simulink subsystem "NAVIGATION"  (R2025b)
settings: Solver=VariableStepAuto  StartTime=0.0  StopTime=10.0  RelTol=1e-3
model mask{refTimePosix=0, omgCelBod=0}
  mask prompts: refTimePosix "Reference time for ECI2ECEF conversion (UTC, Posix) [s]"; omgCelBod "Celestial body angular velocity [rads-1]"
undefined symbols (not defined in the file): simData
libraries: simulink_extras x4, simulink x3, matrix_library x2, aerolibtransform2 x2
settings Model: Creator=antoniohernandez-rodiciomateos  LastModifiedBy=antoniohernandez-rodiciomateos

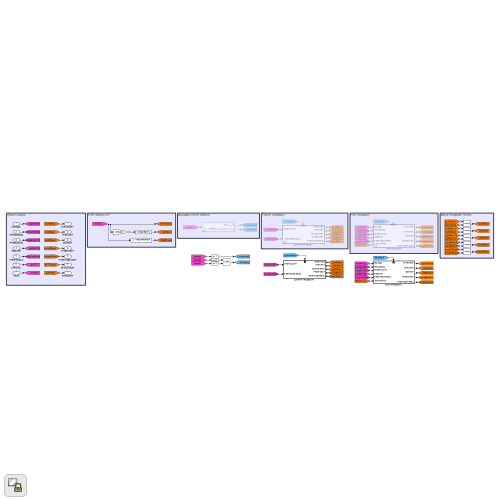
[thumbnail: Simulink's stored preview of the top-level diagram]
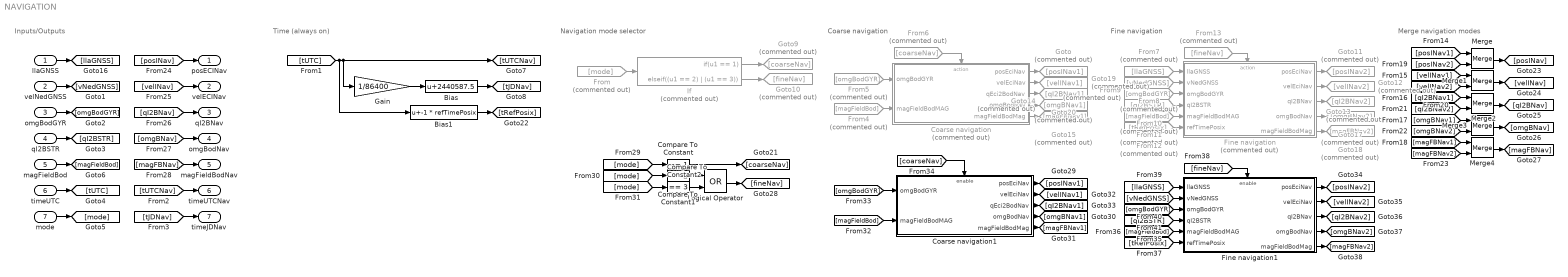
== system NAVIGATION ==
  note: Inputs/Outputs
  note: Time (always on)
  note: Navigation mode selector
  note: Coarse navigation
  note: Fine navigation
  note: Merge navigation modes
  llaGNSS : Inport  PortDimensions=[3 1]
  velNedGNSS : Inport  Port=2  PortDimensions=[3 1]
  omgBodGYR : Inport  Port=3  PortDimensions=[3 1]
  qI2BSTR : Inport  Port=4  PortDimensions=[4 1]
  magFieldBod : Inport  Port=5  PortDimensions=[3 1]
  timeUTC : Inport  Port=6  PortDimensions=[1 1]
  mode : Inport  Port=7  PortDimensions=[1 1]
  Bias : Bias  Bias=2440587.5  SaturateOnIntegerOverflow=off
  Bias1 : Bias  Bias=-1 * refTimePosix  SaturateOnIntegerOverflow=off
  Coarse navigation : Subsystem  Commented=on  TreatAsAtomicUnit=on
  Coarse navigation1 : Subsystem  TreatAsAtomicUnit=on
  Compare To Constant : simulink/Logic and Bit Operations/Compare To Constant  relop===  const=1  OutDataTypeStr=boolean
  Compare To Constant1 : simulink/Logic and Bit Operations/Compare To Constant  relop===  const=2  OutDataTypeStr=boolean
  Compare To Constant2 : simulink/Logic and Bit Operations/Compare To Constant  relop===  const=3  OutDataTypeStr=boolean
  Fine navigation : Subsystem  Commented=on  TreatAsAtomicUnit=on
  Fine navigation1 : Subsystem  TreatAsAtomicUnit=on
  From : From  Commented=on  GotoTag=mode
  From10 : From  Commented=on  GotoTag=qI2BSTR
  From11 : From  Commented=on  GotoTag=magFieldBod
  From12 : From  Commented=on  GotoTag=tRefPosix
  From13 : From  Commented=on  GotoTag=fineNav
  From4 : From  Commented=on  GotoTag=magFieldBod
  From5 : From  Commented=on  GotoTag=omgBodGYR
  From6 : From  Commented=on  GotoTag=coarseNav
  From7 : From  Commented=on  GotoTag=llaGNSS
  From8 : From  Commented=on  GotoTag=vNedGNSS
  From9 : From  Commented=on  GotoTag=omgBodGYR
  Gain : Gain  Gain=1/86400
  Goto : Goto  Commented=on  GotoTag=posINav1
  Goto10 : Goto  Commented=on  GotoTag=fineNav
  Goto11 : Goto  Commented=on  GotoTag=posINav2
  Goto12 : Goto  Commented=on  GotoTag=velINav2
  Goto13 : Goto  Commented=on  GotoTag=qI2BNav2
  Goto14 : Goto  Commented=on  GotoTag=omgBNav1
  Goto15 : Goto  Commented=on  GotoTag=magFBNav1
  Goto17 : Goto  Commented=on  GotoTag=omgBNav2
  Goto18 : Goto  Commented=on  GotoTag=magFBNav2
  Goto19 : Goto  Commented=on  GotoTag=velINav1
  Goto20 : Goto  Commented=on  GotoTag=qI2BNav1
  Goto9 : Goto  Commented=on  GotoTag=coarseNav
  If : If  Commented=on  IfExpression=u1 == 1  ElseIfExpressions=(u1 == 2) | (u1 == 3)  ShowElse=off
  Logical Operator : Logic  Operator=OR  AllPortsSameDT=off  OutDataTypeStr=boolean
  Merge{,1..4} (5 alike) : Merge
  posECINav : Outport  PortDimensions=[3 1]
  velECINav : Outport  Port=2  PortDimensions=[3 1]
  qI2BNav : Outport  Port=3  PortDimensions=[4 1]
  omgBodNav : Outport  Port=4  PortDimensions=[3 1]
  magFieldBodNav : Outport  Port=5  PortDimensions=[3 1]
  timeUTCNav : Outport  Port=6  PortDimensions=[1 1]
  timeJDNav : Outport  Port=7  PortDimensions=[1 1]
  wires:
  llaGNSS/1 -> [llaGNSS]
  velNedGNSS/1 -> [vNedGNSS]
  omgBodGYR/1 -> [omgBodGYR]
  qI2BSTR/1 -> [qI2BSTR]
  timeUTC/1 -> [tUTC]
  mode/1 -> [mode]
  From/1 -> If/1
  magFieldBod/1 -> [magFieldBod]
  [tUTC] -> Bias1/1, Gain/1, [tUTCNav]
  Gain/1 -> Bias/1
  Bias/1 -> [tJDNav]
  [tUTCNav] -> timeUTCNav/1
  [tJDNav] -> timeJDNav/1
  If/1 -> Goto9/1
  If/2 -> Goto10/1
  Bias1/1 -> [tRefPosix]
  [posINav] -> posECINav/1
  [velINav] -> velECINav/1
  [qI2BNav] -> qI2BNav/1
  [omgBNav] -> omgBodNav/1
  [magFBNav] -> magFieldBodNav/1
  From6/1 -> Coarse navigation/Action
  Coarse navigation/2(velEciNav) -> Goto19/1
  Coarse navigation/4(omgBodNav) -> Goto14/1
  Coarse navigation/3(qEci2BodNav) -> Goto20/1
  Coarse navigation/1(posEciNav) -> Goto/1
  Coarse navigation/5(magFieldBodMag) -> Goto15/1
  From5/1 -> Coarse navigation/1(omgBodGYR)
  From4/1 -> Coarse navigation/2(magFieldBodMAG)
  Fine navigation/1(posEciNav) -> Goto11/1
  From10/1 -> Fine navigation/4(qI2BSTR)
  From13/1 -> Fine navigation/Action
  Fine navigation/3(qI2BNav) -> Goto13/1
  Fine navigation/5(magFieldBodMag) -> Goto18/1
  From7/1 -> Fine navigation/1(llaGNSS)
  Fine navigation/4(omgBodNav) -> Goto17/1
  From11/1 -> Fine navigation/5(magFieldBodMAG)
  Fine navigation/2(velEciNav) -> Goto12/1
  From8/1 -> Fine navigation/2(vNedGNSS)
  From9/1 -> Fine navigation/3(omgBodGYR)
  From12/1 -> Fine navigation/6(refTimePosix)
  [qI2BNav2] -> Merge2/2
  Merge2/1 -> [qI2BNav]
  Merge4/1 -> [magFBNav]
  [omgBNav2] -> Merge3/2
  Merge3/1 -> [omgBNav]
  [omgBNav1] -> Merge3/1
  [posINav1] -> Merge/1
  [velINav1] -> Merge1/1
  Merge/1 -> [posINav]
  [velINav2] -> Merge1/2
  [posINav2] -> Merge/2
  [magFBNav1] -> Merge4/1
  [magFBNav2] -> Merge4/2
  Merge1/1 -> [velINav]
  [qI2BNav1] -> Merge2/1
  [mode] -> Compare To Constant/1
  Compare To Constant/1 -> [coarseNav]
  [mode] -> Compare To Constant1/1
  [mode] -> Compare To Constant2/1
  Compare To Constant1/1 -> Logical Operator/1
  Compare To Constant2/1 -> Logical Operator/2
  Logical Operator/1 -> [fineNav]
  Coarse navigation1/1(posEciNav) -> [posINav1]
  Coarse navigation1/2(velEciNav) -> [velINav1]
  Coarse navigation1/3(qEci2BodNav) -> [qI2BNav1]
  Coarse navigation1/4(omgBodNav) -> [omgBNav1]
  Coarse navigation1/5(magFieldBodMag) -> [magFBNav1]
  [omgBodGYR] -> Coarse navigation1/1(omgBodGYR)
  [magFieldBod] -> Coarse navigation1/2(magFieldBodMAG)
  [coarseNav] -> Coarse navigation1/Enable
  [tRefPosix] -> Fine navigation1/6(refTimePosix)
  [qI2BSTR] -> Fine navigation1/4(qI2BSTR)
  Fine navigation1/2(velEciNav) -> [velINav2]
  Fine navigation1/5(magFieldBodMag) -> [magFBNav2]
  Fine navigation1/1(posEciNav) -> [posINav2]
  [magFieldBod] -> Fine navigation1/5(magFieldBodMAG)
  [vNedGNSS] -> Fine navigation1/2(vNedGNSS)
  [fineNav] -> Fine navigation1/Enable
  [llaGNSS] -> Fine navigation1/1(llaGNSS)
  Fine navigation1/3(qI2BNav) -> [qI2BNav2]
  [omgBodGYR] -> Fine navigation1/3(omgBodGYR)
  Fine navigation1/4(omgBodNav) -> [omgBNav2]

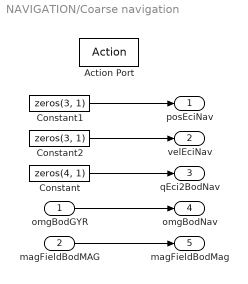
== system NAVIGATION/Coarse navigation ==
  omgBodGYR : Inport  PortDimensions=[3 1]
  magFieldBodMAG : Inport  Port=2  PortDimensions=[3 1]
  Action Port : ActionPort
  Constant : Constant  Value=zeros(4, 1)
  Constant1 : Constant  Value=zeros(3, 1)
  Constant2 : Constant  Value=zeros(3, 1)
  posEciNav : Outport  PortDimensions=[3 1]
  velEciNav : Outport  Port=2  PortDimensions=[3 1]
  qEci2BodNav : Outport  Port=3  PortDimensions=[4 1]
  omgBodNav : Outport  Port=4  PortDimensions=[3 1]
  magFieldBodMag : Outport  Port=5  PortDimensions=[3 1]
  wires:
  omgBodGYR/1 -> omgBodNav/1
  magFieldBodMAG/1 -> magFieldBodMag/1
  Constant/1 -> qEci2BodNav/1
  Constant1/1 -> posEciNav/1
  Constant2/1 -> velEciNav/1

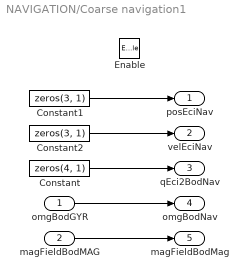
== system NAVIGATION/Coarse navigation1 ==
  omgBodGYR : Inport  PortDimensions=[3 1]
  magFieldBodMAG : Inport  Port=2  PortDimensions=[3 1]
  Enable : EnablePort
  Constant : Constant  Value=zeros(4, 1)
  Constant1 : Constant  Value=zeros(3, 1)
  Constant2 : Constant  Value=zeros(3, 1)
  posEciNav : Outport  PortDimensions=[3 1]
  velEciNav : Outport  Port=2  PortDimensions=[3 1]
  qEci2BodNav : Outport  Port=3  PortDimensions=[4 1]
  omgBodNav : Outport  Port=4  PortDimensions=[3 1]
  magFieldBodMag : Outport  Port=5  PortDimensions=[3 1]
  wires:
  omgBodGYR/1 -> omgBodNav/1
  magFieldBodMAG/1 -> magFieldBodMag/1
  Constant/1 -> qEci2BodNav/1
  Constant1/1 -> posEciNav/1
  Constant2/1 -> velEciNav/1

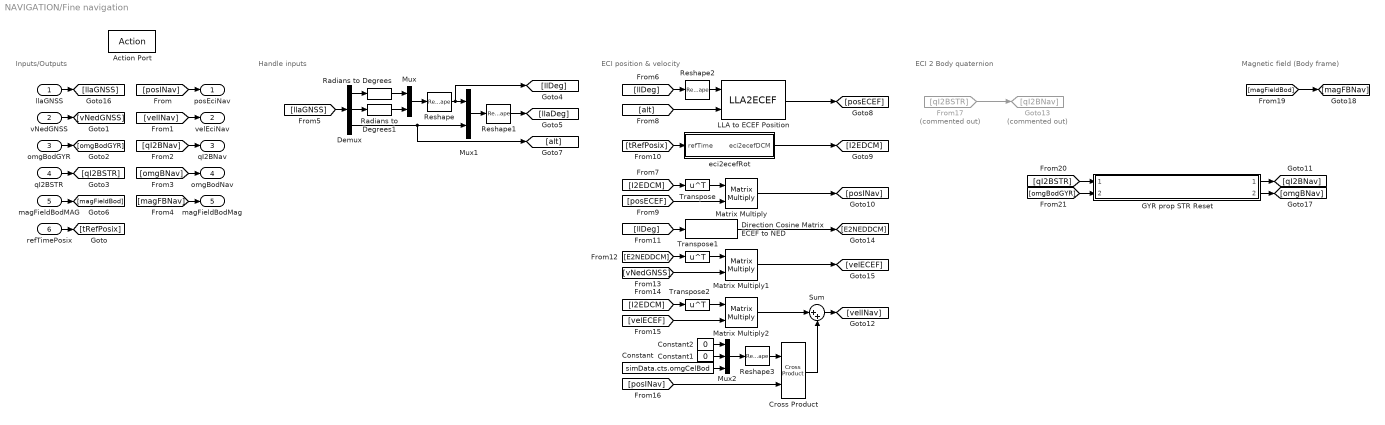
== system NAVIGATION/Fine navigation ==
  note: Inputs/Outputs
  note: Handle inputs
  note: ECI position & velocity
  note: ECI 2 Body quaternion
  note: Magnetic field (Body frame)
  llaGNSS : Inport  PortDimensions=[3 1]
  vNedGNSS : Inport  Port=2  PortDimensions=[3 1]
  omgBodGYR : Inport  Port=3  PortDimensions=[3 1]
  qI2BSTR : Inport  Port=4  PortDimensions=[4 1]
  magFieldBodMAG : Inport  Port=5  PortDimensions=[3 1]
  refTimePosix : Inport  Port=6  PortDimensions=[1 1]
  Action Port : ActionPort
  Constant : Constant  Value=simData.cts.omgCelBod
  Constant1 : Constant  Value=0
  Constant2 : Constant  Value=0
  Cross Product : matrix_library/Cross Product
  Demux : Demux  Outputs=3
  Direction Cosine Matrix ECEF to NED : aerolibtransform2/Direction Cosine Matrix ECEF to NED
  From17 : From  Commented=on  GotoTag=qI2BSTR
  GYR prop STR Reset : Subsystem  ReferencedSubsystem=NAV_GYRO_PROP
  Goto13 : Goto  Commented=on  GotoTag=qI2BNav
  LLA to ECEF Position : LLA2ECEF
  Matrix Multiply : Product  Multiplication=Matrix(*)
  Matrix Multiply1 : Product  Multiplication=Matrix(*)
  Matrix Multiply2 : Product  Multiplication=Matrix(*)
  Mux : Mux  Inputs=2
  Mux1 : Mux  Inputs=2
  Mux2 : Mux  Inputs=3
  Radians to Degrees : simulink_extras/Transformations/Radians to Degrees
  Radians to Degrees1 : simulink_extras/Transformations/Radians to Degrees
  Reshape : Reshape  OutputDimensionality=Column vector (2-D)
  Reshape1 : Reshape  OutputDimensionality=Column vector (2-D)
  Reshape2 : Reshape
  Reshape3 : Reshape  OutputDimensionality=Column vector (2-D)
  Sum : Sum  Inputs=|++
  Transpose : Math  Operator=transpose
  Transpose1 : Math  Operator=transpose
  Transpose2 : Math  Operator=transpose
  eci2ecefRot : Subsystem
  posEciNav : Outport  PortDimensions=[3 1]
  velEciNav : Outport  Port=2  PortDimensions=[3 1]
  qI2BNav : Outport  Port=3  PortDimensions=[4 1]
  omgBodNav : Outport  Port=4  PortDimensions=[3 1]
  magFieldBodMag : Outport  Port=5  PortDimensions=[3 1]
  wires:
  GYR prop STR Reset/2 -> [omgBNav]
  GYR prop STR Reset/1 -> [qI2BNav]
  [omgBodGYR] -> GYR prop STR Reset/2
  [qI2BSTR] -> GYR prop STR Reset/1
  llaGNSS/1 -> [llaGNSS]
  vNedGNSS/1 -> [vNedGNSS]
  omgBodGYR/1 -> [omgBodGYR]
  qI2BSTR/1 -> [qI2BSTR]
  magFieldBodMAG/1 -> [magFieldBod]
  [posINav] -> posEciNav/1
  [velINav] -> velEciNav/1
  [qI2BNav] -> qI2BNav/1
  [omgBNav] -> omgBodNav/1
  [magFBNav] -> magFieldBodMag/1
  Demux/1 -> Radians to Degrees/1
  Radians to Degrees/1 -> Mux/1
  Mux/1 -> Reshape/1
  Demux/2 -> Radians to Degrees1/1
  Radians to Degrees1/1 -> Mux/2
  Reshape/1 -> [llDeg], Mux1/1
  Demux/3 -> [alt], Mux1/2
  Mux1/1 -> Reshape1/1
  [llaGNSS] -> Demux/1
  Reshape1/1 -> [llaDeg]
  [tRefPosix] -> eci2ecefRot/1(refTime)
  [llDeg] -> Reshape2/1
  Reshape2/1 -> LLA to ECEF Position/1
  [alt] -> LLA to ECEF Position/2
  LLA to ECEF Position/1 -> [posECEF]
  refTimePosix/1 -> [tRefPosix]
  eci2ecefRot/1(eci2ecefDCM) -> [I2EDCM]
  [I2EDCM] -> Transpose/1
  Transpose/1 -> Matrix Multiply/1
  [posECEF] -> Matrix Multiply/2
  Matrix Multiply/1 -> [posINav]
  [llDeg] -> Direction Cosine Matrix ECEF to NED/1
  Direction Cosine Matrix ECEF to NED/1 -> [E2NEDDCM]
  [E2NEDDCM] -> Transpose1/1
  Transpose1/1 -> Matrix Multiply1/1
  [vNedGNSS] -> Matrix Multiply1/2
  Matrix Multiply1/1 -> [velECEF]
  Constant/1 -> Mux2/3
  Constant2/1 -> Mux2/1
  Mux2/1 -> Reshape3/1
  Constant1/1 -> Mux2/2
  [I2EDCM] -> Transpose2/1
  [velECEF] -> Matrix Multiply2/2
  Transpose2/1 -> Matrix Multiply2/1
  Matrix Multiply2/1 -> Sum/1
  Reshape3/1 -> Cross Product/1
  [posINav] -> Cross Product/2
  Cross Product/1 -> Sum/2
  Sum/1 -> [velINav]
  From17/1 -> Goto13/1
  [magFieldBod] -> [magFBNav]

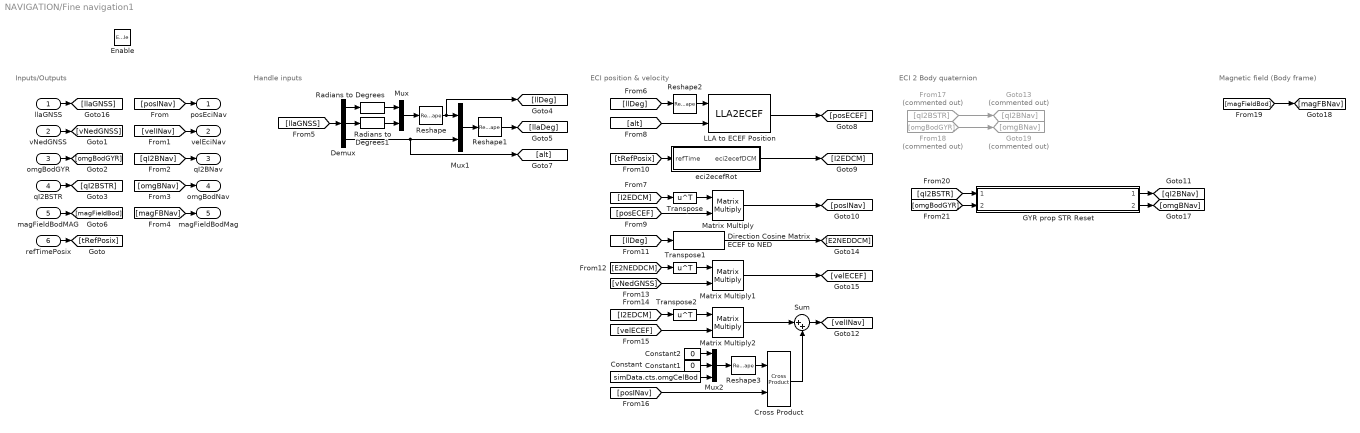
== system NAVIGATION/Fine navigation1 ==
  note: Inputs/Outputs
  note: Handle inputs
  note: ECI position & velocity
  note: ECI 2 Body quaternion
  note: Magnetic field (Body frame)
  llaGNSS : Inport  PortDimensions=[3 1]
  vNedGNSS : Inport  Port=2  PortDimensions=[3 1]
  omgBodGYR : Inport  Port=3  PortDimensions=[3 1]
  qI2BSTR : Inport  Port=4  PortDimensions=[4 1]
  magFieldBodMAG : Inport  Port=5  PortDimensions=[3 1]
  refTimePosix : Inport  Port=6  PortDimensions=[1 1]
  Enable : EnablePort
  Constant : Constant  Value=simData.cts.omgCelBod
  Constant1 : Constant  Value=0
  Constant2 : Constant  Value=0
  Cross Product : matrix_library/Cross Product
  Demux : Demux  Outputs=3
  Direction Cosine Matrix ECEF to NED : aerolibtransform2/Direction Cosine Matrix ECEF to NED
  From17 : From  Commented=on  GotoTag=qI2BSTR
  From18 : From  Commented=on  GotoTag=omgBodGYR
  GYR prop STR Reset : Subsystem  ReferencedSubsystem=NAV_GYRO_PROP
  Goto13 : Goto  Commented=on  GotoTag=qI2BNav
  Goto19 : Goto  Commented=on  GotoTag=omgBNav
  LLA to ECEF Position : LLA2ECEF
  Matrix Multiply : Product  Multiplication=Matrix(*)
  Matrix Multiply1 : Product  Multiplication=Matrix(*)
  Matrix Multiply2 : Product  Multiplication=Matrix(*)
  Mux : Mux  Inputs=2
  Mux1 : Mux  Inputs=2
  Mux2 : Mux  Inputs=3
  Radians to Degrees : simulink_extras/Transformations/Radians to Degrees
  Radians to Degrees1 : simulink_extras/Transformations/Radians to Degrees
  Reshape : Reshape  OutputDimensionality=Column vector (2-D)
  Reshape1 : Reshape  OutputDimensionality=Column vector (2-D)
  Reshape2 : Reshape
  Reshape3 : Reshape  OutputDimensionality=Column vector (2-D)
  Sum : Sum  Inputs=|++
  Transpose : Math  Operator=transpose
  Transpose1 : Math  Operator=transpose
  Transpose2 : Math  Operator=transpose
  eci2ecefRot : Subsystem
  posEciNav : Outport  PortDimensions=[3 1]
  velEciNav : Outport  Port=2  PortDimensions=[3 1]
  qI2BNav : Outport  Port=3  PortDimensions=[4 1]
  omgBodNav : Outport  Port=4  PortDimensions=[3 1]
  magFieldBodMag : Outport  Port=5  PortDimensions=[3 1]
  wires:
  llaGNSS/1 -> [llaGNSS]
  vNedGNSS/1 -> [vNedGNSS]
  omgBodGYR/1 -> [omgBodGYR]
  qI2BSTR/1 -> [qI2BSTR]
  magFieldBodMAG/1 -> [magFieldBod]
  [posINav] -> posEciNav/1
  [velINav] -> velEciNav/1
  [qI2BNav] -> qI2BNav/1
  [omgBNav] -> omgBodNav/1
  [magFBNav] -> magFieldBodMag/1
  Demux/1 -> Radians to Degrees/1
  Radians to Degrees/1 -> Mux/1
  Mux/1 -> Reshape/1
  Demux/2 -> Radians to Degrees1/1
  Radians to Degrees1/1 -> Mux/2
  Reshape/1 -> [llDeg], Mux1/1
  Demux/3 -> [alt], Mux1/2
  Mux1/1 -> Reshape1/1
  [llaGNSS] -> Demux/1
  Reshape1/1 -> [llaDeg]
  [tRefPosix] -> eci2ecefRot/1(refTime)
  [llDeg] -> Reshape2/1
  Reshape2/1 -> LLA to ECEF Position/1
  [alt] -> LLA to ECEF Position/2
  LLA to ECEF Position/1 -> [posECEF]
  refTimePosix/1 -> [tRefPosix]
  eci2ecefRot/1(eci2ecefDCM) -> [I2EDCM]
  [I2EDCM] -> Transpose/1
  Transpose/1 -> Matrix Multiply/1
  [posECEF] -> Matrix Multiply/2
  Matrix Multiply/1 -> [posINav]
  [llDeg] -> Direction Cosine Matrix ECEF to NED/1
  Direction Cosine Matrix ECEF to NED/1 -> [E2NEDDCM]
  [E2NEDDCM] -> Transpose1/1
  Transpose1/1 -> Matrix Multiply1/1
  [vNedGNSS] -> Matrix Multiply1/2
  Matrix Multiply1/1 -> [velECEF]
  Constant/1 -> Mux2/3
  Constant2/1 -> Mux2/1
  Mux2/1 -> Reshape3/1
  Constant1/1 -> Mux2/2
  [I2EDCM] -> Transpose2/1
  [velECEF] -> Matrix Multiply2/2
  Transpose2/1 -> Matrix Multiply2/1
  Matrix Multiply2/1 -> Sum/1
  Reshape3/1 -> Cross Product/1
  [posINav] -> Cross Product/2
  Cross Product/1 -> Sum/2
  Sum/1 -> [velINav]
  From17/1 -> Goto13/1
  [magFieldBod] -> [magFBNav]
  [omgBodGYR] -> GYR prop STR Reset/2
  GYR prop STR Reset/1 -> [qI2BNav]
  GYR prop STR Reset/2 -> [omgBNav]
  [qI2BSTR] -> GYR prop STR Reset/1
  From18/1 -> Goto19/1

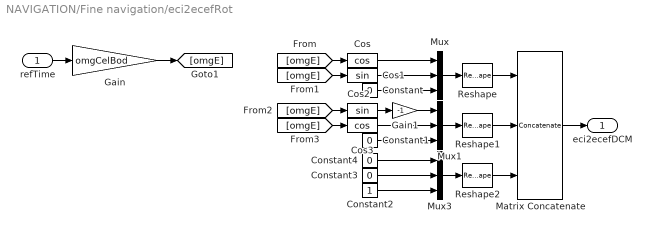
== system NAVIGATION/Fine navigation/eci2ecefRot ==
  refTime : Inport  PortDimensions=[1 1]
  Constant{,1,3..4} (4 alike) : Constant  Value=0
  Constant2 : Constant
  Cos : Trigonometry  Operator=cos
  Cos1 : Trigonometry
  Cos2 : Trigonometry
  Cos3 : Trigonometry  Operator=cos
  Gain : Gain  Gain=omgCelBod
  Gain1 : Gain  Gain=-1
  Matrix Concatenate : Concatenate  NumInputs=3  Mode=Multidimensional array
  Mux : Mux  Inputs=3
  Mux1 : Mux  Inputs=3
  Mux3 : Mux  Inputs=3
  Reshape : Reshape  OutputDimensionality=Row vector (2-D)
  Reshape1 : Reshape  OutputDimensionality=Row vector (2-D)
  Reshape2 : Reshape  OutputDimensionality=Row vector (2-D)
  eci2ecefDCM : Outport  PortDimensions=[3 3]
  wires:
  Matrix Concatenate/1 -> eci2ecefDCM/1
  Reshape2/1 -> Matrix Concatenate/3
  Reshape1/1 -> Matrix Concatenate/2
  Constant3/1 -> Mux3/2
  Constant2/1 -> Mux3/3
  Mux3/1 -> Reshape2/1
  Constant4/1 -> Mux3/1
  Gain1/1 -> Mux1/1
  Cos2/1 -> Gain1/1
  [omgE] -> Cos2/1
  Constant1/1 -> Mux1/3
  [omgE] -> Cos3/1
  Cos3/1 -> Mux1/2
  Mux1/1 -> Reshape1/1
  [omgE] -> Cos1/1
  [omgE] -> Cos/1
  Gain/1 -> [omgE]
  refTime/1 -> Gain/1
  Mux/1 -> Reshape/1
  Cos1/1 -> Mux/2
  Constant/1 -> Mux/3
  Cos/1 -> Mux/1
  Reshape/1 -> Matrix Concatenate/1

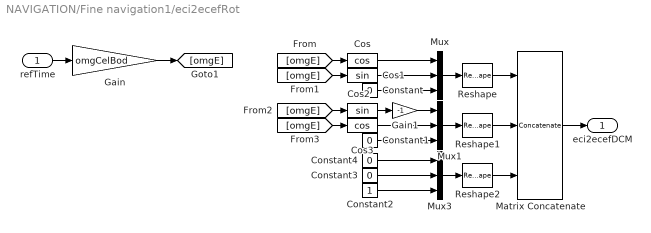
== system NAVIGATION/Fine navigation1/eci2ecefRot ==
  refTime : Inport  PortDimensions=[1 1]
  Constant{,1,3..4} (4 alike) : Constant  Value=0
  Constant2 : Constant
  Cos : Trigonometry  Operator=cos
  Cos1 : Trigonometry
  Cos2 : Trigonometry
  Cos3 : Trigonometry  Operator=cos
  Gain : Gain  Gain=omgCelBod
  Gain1 : Gain  Gain=-1
  Matrix Concatenate : Concatenate  NumInputs=3  Mode=Multidimensional array
  Mux : Mux  Inputs=3
  Mux1 : Mux  Inputs=3
  Mux3 : Mux  Inputs=3
  Reshape : Reshape  OutputDimensionality=Row vector (2-D)
  Reshape1 : Reshape  OutputDimensionality=Row vector (2-D)
  Reshape2 : Reshape  OutputDimensionality=Row vector (2-D)
  eci2ecefDCM : Outport  PortDimensions=[3 3]
  wires:
  Matrix Concatenate/1 -> eci2ecefDCM/1
  Reshape2/1 -> Matrix Concatenate/3
  Reshape1/1 -> Matrix Concatenate/2
  Constant3/1 -> Mux3/2
  Constant2/1 -> Mux3/3
  Mux3/1 -> Reshape2/1
  Constant4/1 -> Mux3/1
  Gain1/1 -> Mux1/1
  Cos2/1 -> Gain1/1
  [omgE] -> Cos2/1
  Constant1/1 -> Mux1/3
  [omgE] -> Cos3/1
  Cos3/1 -> Mux1/2
  Mux1/1 -> Reshape1/1
  [omgE] -> Cos1/1
  [omgE] -> Cos/1
  Gain/1 -> [omgE]
  refTime/1 -> Gain/1
  Mux/1 -> Reshape/1
  Cos1/1 -> Mux/2
  Constant/1 -> Mux/3
  Cos/1 -> Mux/1
  Reshape/1 -> Matrix Concatenate/1
